simulink model "Controller"  (R2020b)
settings: Solver=FixedStepAuto  StartTime=0.0  StopTime=16.9  RelTol=1e-3
settings Model: Creator=michaelgiancola  LastModifiedBy=michaelgiancola

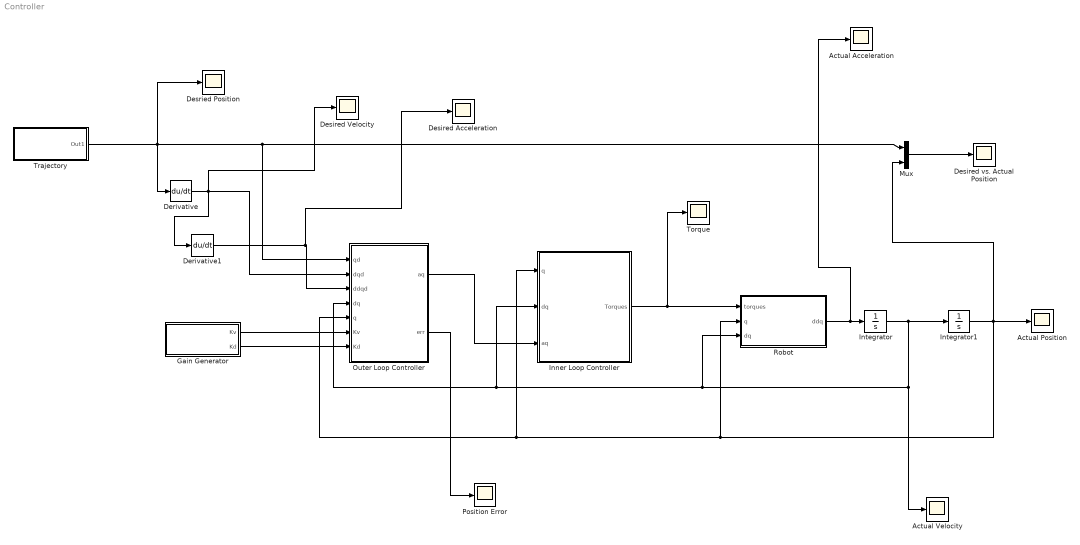
== system Controller ==
  Actual Acceleration : Scope
  Actual Position : Scope
  Actual Velocity : Scope
  Derivative : Derivative
  Derivative1 : Derivative
  Desired Acceleration : Scope
  Desired Velocity : Scope
  Desired vs. Actual Position : Scope
  Desried Position : Scope
  Gain Generator : Subsystem
  Inner Loop Controller : MATLAB Function  TreatAsAtomicUnit=on
  Integrator : Integrator  InitialCondition=[0,0,0]
  Integrator1 : Integrator  InitialCondition=[0,0,0]
  Mux : Mux  Inputs=2
  Outer Loop Controller : MATLAB Function  TreatAsAtomicUnit=on
  Position Error : Scope
  Robot : MATLAB Function  TreatAsAtomicUnit=on
  Torque : Scope
  Trajectory : Subsystem
  wires:
  Gain Generator/2(Kd) -> Outer Loop Controller/7(Kd)
  Trajectory/1(Out1) -> Derivative/1, Desried Position/1, Outer Loop Controller/1(qd), Mux/1
  Gain Generator/1(Kv) -> Outer Loop Controller/6(Kv)
  Derivative1/1 -> Desired Acceleration/1, Outer Loop Controller/3(ddqd)
  Derivative/1 -> Desired Velocity/1, Derivative1/1, Outer Loop Controller/2(dqd)
  Outer Loop Controller/1(aq) -> Inner Loop Controller/3(aq)
  Robot/1(ddq) -> Actual Acceleration/1, Integrator/1
  Integrator/1 -> Robot/3(dq), Inner Loop Controller/2(dq), Outer Loop Controller/4(dq), Actual Velocity/1, Integrator1/1
  Inner Loop Controller/1(Torques) -> Robot/1(torques), Torque/1
  Integrator1/1 -> Mux/2, Inner Loop Controller/1(q), Outer Loop Controller/5(q), Robot/2(q), Actual Position/1
  Outer Loop Controller/2(err) -> Position Error/1
  Mux/1 -> Desired vs. Actual Position/1

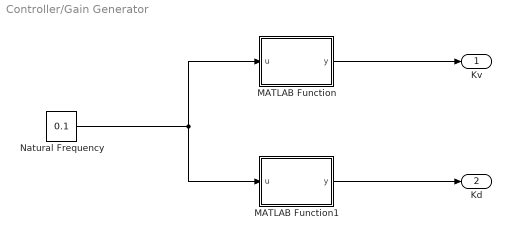
== system Controller/Gain Generator ==
  MATLAB Function : MATLAB Function  TreatAsAtomicUnit=on
  MATLAB Function1 : MATLAB Function  TreatAsAtomicUnit=on
  Natural Frequency : Constant  Value=0.1
  Kv : Outport
  Kd : Outport  Port=2
  wires:
  Natural Frequency/1 -> MATLAB Function/1(u), MATLAB Function1/1(u)
  MATLAB Function1/1(y) -> Kd/1
  MATLAB Function/1(y) -> Kv/1

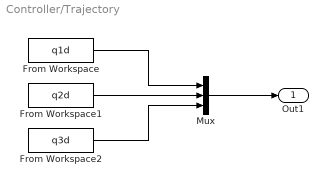
== system Controller/Trajectory ==
  From Workspace : FromWorkspace  VariableName=q1d
  From Workspace1 : FromWorkspace  VariableName=q2d
  From Workspace2 : FromWorkspace  VariableName=q3d
  Mux : Mux  Inputs=3
  Out1 : Outport
  wires:
  Mux/1 -> Out1/1
  From Workspace1/1 -> Mux/2
  From Workspace/1 -> Mux/1
  From Workspace2/1 -> Mux/3

== matlab function Controller/Inner Loop Controller ==
  data: q input; dq input; aq input; Torques output
%Michael Giancola
%Automated BlackJack Dealing Arm
%Inverse Dynamic Equations of motion
%ddq = dynamicEqns(q, dq, aq) 
%Returns a matrix of required torque values for each joint
%these inverse dynamic equations take in aq as the new acceleration inputs
%Date: Dec 4, 2020

function Torques  = inverseDyn(q,dq,aq)

theta1 = q(1);
theta2 = q(2);
theta3 = q(3);
dtheta1 = dq(1);
dtheta2 = dq(2);
dtheta3 = dq(3);
ddtheta1 = aq(1);
ddtheta2 = aq(2);
ddtheta3 = aq(3);

%Inverse Dynamic Eqns of motion found using Euler-Lagrange
Torq1 = ddtheta1*((1424533*cos(2*theta2 + theta3))/4 + (815624558777204737*cos(2*theta2))/1717986918400 + (203792294069927937*cos(2*theta2 + 2*theta3))/1717986918400 + (1424533*cos(theta3))/4 + 32855125699743187007/54975581388800) - 2*dtheta1*dtheta3*((1424533*sin(2*theta2 + theta3))/4 + (203792294069927937*sin(2*theta2 + 2*theta3))/858993459200 + (1424533*sin(theta3))/4) - 2*dtheta1*dtheta2*((1424533*sin(2*theta2 + theta3))/2 + (815624558777204737*sin(2*theta2))/858993459200 + (203792294069927937*sin(2*theta2 + 2*theta3))/858993459200);
 
Torq2 = ((1424533*sin(2*theta2 + theta3))/2 + (815624558777204737*sin(2*theta2))/858993459200 + (203792294069927937*sin(2*theta2 + 2*theta3))/858993459200)*dtheta1^2 + (343596100481210885*cos(theta2 + theta3))/137438953472 + (1030788301443632655*cos(theta2))/137438953472 - (1424533*dtheta3^2*sin(theta3))/2 + ddtheta2*((1424533*cos(theta3))/2 + 20400472916534231/17179869184) + ddtheta3*((1424533*cos(theta3))/4 + 8163827622388695/34359738368) - 1424533*dtheta2*dtheta3*sin(theta3);
 
Torq3 = ((1424533*sin(2*theta2 + theta3))/4 + (203792294069927937*sin(2*theta2 + 2*theta3))/858993459200 + (1424533*sin(theta3))/4)*dtheta1^2 + (1424533*sin(theta3)*dtheta2^2)/2 + (8163827622388695*ddtheta3)/34359738368 + (343596100481210885*cos(theta2 + theta3))/137438953472 + ddtheta2*((1424533*cos(theta3))/4 + 8163827622388695/34359738368);

Torques = [Torq1; Torq2; Torq3];

end

== matlab function Controller/Outer Loop Controller ==
  data: qd input; aq output; dqd input; ddqd input; dq input; q input; Kv input; Kd input; err output
%Michael Giancola
%Automated BlackJack Dealing Arm
%computes the outer loop controller of the control system
%calculates the new input aq for each joint which helps linearize the system
%Date: Dec 4, 2020

function [aq,err] = control(qd,dqd,ddqd,dq,q,Kv,Kd)

aq = ddqd-Kd*(q-qd)-Kv*(dq-dqd);
err = [qd-q];

== matlab function Controller/Gain Generator/MATLAB Function ==
  data: u input; y output
%Michael Giancola
%Automated BlackJack Dealing Arm
%computes derivative gain using natural freq
%Date: Dec 4, 2020

function y = dergain(u)

I = eye(3);
y = I*(2*u);

== matlab function Controller/Gain Generator/MATLAB Function1 ==
  data: u input; y output
%Michael Giancola
%Automated BlackJack Dealing Arm
%computes position gain using natural freq
%Date: Dec 4, 2020

function y = posgain(u)

I = eye(3);
y = I*(u^2);

== matlab function Controller/Robot ==
  data: torques input; ddq output; q input; dq input
%Michael Giancola
%Automated BlackJack Dealing Arm
%Forward Dynamics
%ddq = forwardDyn(torques, q, dq) 
%ddq is a matrix of angular accelerations for each joint
%Date: Dec 4, 2020

function ddq = forwardDyn(torques, q, dq)

theta1 = q(1);
theta2 = q(2);
theta3 = q(3);
dtheta1 = dq(1);
dtheta2 = dq(2);
dtheta3 = dq(3);
Torq1 = torques(1);
Torq2 = torques(2);
Torq3 = torques(3);

%Forward dynamics equations
ddtheta1 = (Torq1 + 2*dtheta1*dtheta3*((1424533*sin(2*theta2 + theta3))/4 + (47449091*sin(2*theta2 + 2*theta3))/200 + (1424533*sin(theta3))/4) + 2*dtheta1*dtheta2*((1424533*sin(2*theta2 + theta3))/2 + (189902391*sin(2*theta2))/200 + (47449091*sin(2*theta2 + 2*theta3))/200))/((1424533*cos(2*theta2 + theta3))/4 + (189902391*cos(2*theta2))/400 + (47449091*cos(2*theta2 + 2*theta3))/400 + (1424533*cos(theta3))/4 + 5133613390584873/8589934592);

ddtheta2 = -(128*(54786519763032628789248000*Torq2 - 54786519763032628789248000*Torq3 + 102648037256839986627276177408000*cos(theta2 + 2*theta3) - 308249326422879392341591736117625*cos(theta2) + 19511301339398039946758455296000*dtheta1^2*sin(theta3) + 39022602678796079893516910592000*dtheta2^2*sin(theta3) + 39022602678796079893516910592000*dtheta3^2*sin(theta3) - 9770152838562466117526837264384*dtheta1^2*sin(2*theta2 + theta3) - 37397849232498121991343508029440*dtheta1^2*sin(2*theta2) + 14622606255345126099124643430400*dtheta1^2*sin(2*theta3) + 29245212510690252198249286860800*dtheta2^2*sin(2*theta3) - 82118736486105277163110400*Torq3*cos(theta3) + 14622606255345126099124643430400*dtheta1^2*sin(2*theta2 + 2*theta3) + 9741148500835573829231618031616*dtheta1^2*sin(2*theta2 + 3*theta3) + 78045205357592159787033821184000*dtheta2*dtheta3*sin(theta3)))/(25*(74867744027367045627518174363648*cos(2*theta3) - 191576063136145552594161316447807));

ddtheta3 = (128*(54786519763032628789248000*Torq2 - 273810512498275825326489600*Torq3 - 307944111770519959881828532224000*cos(theta2 - theta3) + 102648037256839986627276177408000*cos(theta2 + 2*theta3) + 239613825150079813171205502868125*cos(theta2 + theta3) - 308249326422879392341591736117625*cos(theta2) + 97513027700176589069955052339200*dtheta1^2*sin(theta3) + 195026055400353178139910104678400*dtheta2^2*sin(theta3) + 39022602678796079893516910592000*dtheta3^2*sin(theta3) + 29245212510690256978188854886400*dtheta1^2*sin(2*theta2 + theta3) - 52020455487843248090468151459840*dtheta1^2*sin(2*theta2) + 29245212510690252198249286860800*dtheta1^2*sin(2*theta3) + 58490425021380504396498573721600*dtheta2^2*sin(2*theta3) + 29245212510690252198249286860800*dtheta3^2*sin(2*theta3) + 82118736486105277163110400*Torq2*cos(theta3) - 164237472972210554326220800*Torq3*cos(theta3) - 38986361011525826027480904892416*dtheta1^2*sin(2*theta2 - theta3) + 51962446812389466698132307836928*dtheta1^2*sin(2*theta2 + 2*theta3) + 9741148500835573829231618031616*dtheta1^2*sin(2*theta2 + 3*theta3) + 78045205357592159787033821184000*dtheta2*dtheta3*sin(theta3) + 58490425021380504396498573721600*dtheta2*dtheta3*sin(2*theta3)))/(25*(74867744027367045627518174363648*cos(2*theta3) - 191576063136145552594161316447807));

ddq = [ddtheta1; ddtheta2; ddtheta3];

end
